simulink model "controller_simulation"  (R2017b)
settings: Solver=FixedStepAuto  StartTime=0.0  StopTime=10  FixedStep=0.01  RelTol=1e-3
values from neighbouring files (symbols this model uses):
  g = sym(zeros(length(d),1))    [kinematic_dynamic.m]    (also in simplifyG.m = g*49/5)
  m = [0 0 m1 0 0 0 0 m2]    [kinematic_dynamic.m]
libraries: simulink x6
settings Model: Creator=Ufuk  LastModifiedBy=Ufuk

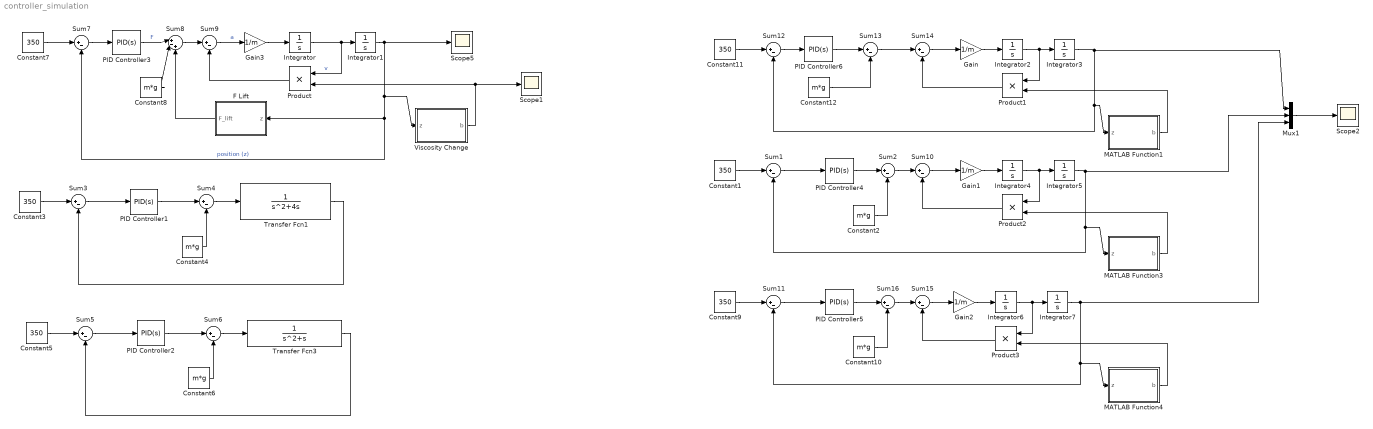
== system controller_simulation ==
  Constant{1,3,5,7,9,11} (6 alike) : Constant  Value=350
  Constant{2,4,6,8,10,12} (6 alike) : Constant  Value=m*g
  F Lift : MATLAB Function  TreatAsAtomicUnit=on
  Gain{,1..3} (4 alike) : Gain  Gain=1/m
  Integrator{,1..7} (8 alike) : Integrator
  MATLAB Function1 : MATLAB Function  TreatAsAtomicUnit=on
  MATLAB Function3 : MATLAB Function  TreatAsAtomicUnit=on
  MATLAB Function4 : MATLAB Function  TreatAsAtomicUnit=on
  Mux1 : Mux  Inputs=3
  PID Controller{1..3,6} (4 alike) : simulink/Continuous/PID Controller  Controller=PID  TimeDomain=Continuous-time  SampleTime=-1  IntegratorMethod=Forward Euler  FilterMethod=Forward Euler  Form=Parallel  UseFilter=on  ControllerParametersSource=internal  P=20  I=0  D=0  N=100  InitialConditionSource=internal  InitialConditionForIntegrator=0  InitialConditionForFilter=0  ExternalReset=none  LimitOutput=off  UpperSaturationLimit=inf  LowerSaturationLimit=-inf  LinearizeAsGain=on  AntiWindupMode=none  Kb=1  TrackingMode=off  Kt=1  PParamMin=[]  PParamMax=[]  IParamMin=[]  IParamMax=[]  DParamMin=[]  DParamMax=[]  NParamMin=[]  NParamMax=[]  KbParamMin=[]  KbParamMax=[]  KtParamMin=[]  KtParamMax=[]  POutMin=[]  POutMax=[]  IOutMin=[]  IOutMax=[]  DOutMin=[]  DOutMax=[]  NOutMin=[]  NOutMax=[]  KbOutMin=[]  KbOutMax=[]  KtOutMin=[]  KtOutMax=[]  IntegratorOutMin=[]  IntegratorOutMax=[]  FilterOutMin=[]  FilterOutMax=[]  SumOutMin=[]  SumOutMax=[]  SumI1OutMin=[]  SumI1OutMax=[]  SumI2OutMin=[]  SumI2OutMax=[]  SumI3OutMin=[]  SumI3OutMax=[]  SumDOutMin=[]  SumDOutMax=[]  SaturationOutMin=[]  SaturationOutMax=[]  IntegratorContinuousStateAttributes=''  IntegratorStateMustResolveToSignalObject=off  IntegratorRTWStateStorageClass=Auto  FilterContinuousStateAttributes=''  FilterStateMustResolveToSignalObject=off  FilterRTWStateStorageClass=Auto  DifferentiatorICPrevScaledInput=0  DifferentiatorOutMin=[]  DifferentiatorOutMax=[]  InitialConditionSetting=State (most efficient)  FilterDiffOutCoefMin=[]  FilterDiffOutCoefMax=[]  SumDenOutMin=[]  SumDenOutMax=[]  SumNumOutMin=[]  SumNumOutMax=[]  ReciprocalOutMin=[]  ReciprocalOutMax=[]  DivideOutMin=[]  DivideOutMax=[]  TunerSelectOption=Transfer Function Based (PID Tuner App)
  PID Controller4 : simulink/Continuous/PID Controller  Controller=PID  TimeDomain=Continuous-time  SampleTime=-1  IntegratorMethod=Forward Euler  FilterMethod=Forward Euler  Form=Parallel  UseFilter=on  ControllerParametersSource=internal  P=15  I=2  D=0  N=100  InitialConditionSource=internal  InitialConditionForIntegrator=0  InitialConditionForFilter=0  ExternalReset=none  LimitOutput=off  UpperSaturationLimit=inf  LowerSaturationLimit=-inf  LinearizeAsGain=on  AntiWindupMode=none  Kb=1  TrackingMode=off  Kt=1  PParamMin=[]  PParamMax=[]  IParamMin=[]  IParamMax=[]  DParamMin=[]  DParamMax=[]  NParamMin=[]  NParamMax=[]  KbParamMin=[]  KbParamMax=[]  KtParamMin=[]  KtParamMax=[]  POutMin=[]  POutMax=[]  IOutMin=[]  IOutMax=[]  DOutMin=[]  DOutMax=[]  NOutMin=[]  NOutMax=[]  KbOutMin=[]  KbOutMax=[]  KtOutMin=[]  KtOutMax=[]  IntegratorOutMin=[]  IntegratorOutMax=[]  FilterOutMin=[]  FilterOutMax=[]  SumOutMin=[]  SumOutMax=[]  SumI1OutMin=[]  SumI1OutMax=[]  SumI2OutMin=[]  SumI2OutMax=[]  SumI3OutMin=[]  SumI3OutMax=[]  SumDOutMin=[]  SumDOutMax=[]  SaturationOutMin=[]  SaturationOutMax=[]  IntegratorContinuousStateAttributes=''  IntegratorStateMustResolveToSignalObject=off  IntegratorRTWStateStorageClass=Auto  FilterContinuousStateAttributes=''  FilterStateMustResolveToSignalObject=off  FilterRTWStateStorageClass=Auto  DifferentiatorICPrevScaledInput=0  DifferentiatorOutMin=[]  DifferentiatorOutMax=[]  InitialConditionSetting=State (most efficient)  FilterDiffOutCoefMin=[]  FilterDiffOutCoefMax=[]  SumDenOutMin=[]  SumDenOutMax=[]  SumNumOutMin=[]  SumNumOutMax=[]  ReciprocalOutMin=[]  ReciprocalOutMax=[]  DivideOutMin=[]  DivideOutMax=[]  TunerSelectOption=Transfer Function Based (PID Tuner App)
  PID Controller5 : simulink/Continuous/PID Controller  Controller=PID  TimeDomain=Continuous-time  SampleTime=-1  IntegratorMethod=Forward Euler  FilterMethod=Forward Euler  Form=Parallel  UseFilter=on  ControllerParametersSource=internal  P=15  I=2  D=1  N=100  InitialConditionSource=internal  InitialConditionForIntegrator=0  InitialConditionForFilter=0  ExternalReset=none  LimitOutput=off  UpperSaturationLimit=inf  LowerSaturationLimit=-inf  LinearizeAsGain=on  AntiWindupMode=none  Kb=1  TrackingMode=off  Kt=1  PParamMin=[]  PParamMax=[]  IParamMin=[]  IParamMax=[]  DParamMin=[]  DParamMax=[]  NParamMin=[]  NParamMax=[]  KbParamMin=[]  KbParamMax=[]  KtParamMin=[]  KtParamMax=[]  POutMin=[]  POutMax=[]  IOutMin=[]  IOutMax=[]  DOutMin=[]  DOutMax=[]  NOutMin=[]  NOutMax=[]  KbOutMin=[]  KbOutMax=[]  KtOutMin=[]  KtOutMax=[]  IntegratorOutMin=[]  IntegratorOutMax=[]  FilterOutMin=[]  FilterOutMax=[]  SumOutMin=[]  SumOutMax=[]  SumI1OutMin=[]  SumI1OutMax=[]  SumI2OutMin=[]  SumI2OutMax=[]  SumI3OutMin=[]  SumI3OutMax=[]  SumDOutMin=[]  SumDOutMax=[]  SaturationOutMin=[]  SaturationOutMax=[]  IntegratorContinuousStateAttributes=''  IntegratorStateMustResolveToSignalObject=off  IntegratorRTWStateStorageClass=Auto  FilterContinuousStateAttributes=''  FilterStateMustResolveToSignalObject=off  FilterRTWStateStorageClass=Auto  DifferentiatorICPrevScaledInput=0  DifferentiatorOutMin=[]  DifferentiatorOutMax=[]  InitialConditionSetting=State (most efficient)  FilterDiffOutCoefMin=[]  FilterDiffOutCoefMax=[]  SumDenOutMin=[]  SumDenOutMax=[]  SumNumOutMin=[]  SumNumOutMax=[]  ReciprocalOutMin=[]  ReciprocalOutMax=[]  DivideOutMin=[]  DivideOutMax=[]  TunerSelectOption=Transfer Function Based (PID Tuner App)
  Product{,1..3} (4 alike) : Product
  Scope1 : Scope
  Scope2 : Scope
  Scope5 : Scope
  Sum{1..7,9..16} (15 alike) : Sum  Inputs=|+-
  Sum8 : Sum  Inputs=|+-+
  Transfer Fcn1 : TransferFcn  Denominator=[1 4 0]
  Transfer Fcn3 : TransferFcn  Denominator=[1 1 0]
  Viscosity Change : MATLAB Function  TreatAsAtomicUnit=on
  wires:
  Transfer Fcn1/1 -> Sum3/2
  Product/1 -> Sum9/2
  Sum6/1 -> Transfer Fcn3/1
  PID Controller2/1 -> Sum6/1
  Sum5/1 -> PID Controller2/1
  Viscosity Change/1(b) -> Product/2, Scope1/1
  Sum8/1 -> Sum9/1
  Integrator/1 -> Product/1, Integrator1/1  "v"
  Sum9/1 -> Gain3/1  "a"
  Integrator1/1 -> Scope5/1, F Lift/1(z), Sum7/2, Viscosity Change/1(z)  "position (z)"
  Sum3/1 -> PID Controller1/1
  Sum7/1 -> PID Controller3/1
  Constant6/1 -> Sum6/2
  Constant8/1 -> Sum8/2
  Constant3/1 -> Sum3/1
  PID Controller1/1 -> Sum4/1
  Constant4/1 -> Sum4/2
  Constant7/1 -> Sum7/1
  Sum4/1 -> Transfer Fcn1/1
  Transfer Fcn3/1 -> Sum5/2
  PID Controller3/1 -> Sum8/1  "F"
  Constant5/1 -> Sum5/1
  MATLAB Function1/1(b) -> Product1/2
  Constant12/1 -> Sum13/2
  Sum13/1 -> Sum14/1
  Product1/1 -> Sum14/2
  Integrator2/1 -> Product1/1, Integrator3/1
  Integrator3/1 -> Mux1/1, MATLAB Function1/1(z), Sum12/2
  Mux1/1 -> Scope2/1
  Sum12/1 -> PID Controller6/1
  Constant11/1 -> Sum12/1
  PID Controller6/1 -> Sum13/1
  Sum14/1 -> Gain/1
  PID Controller4/1 -> Sum2/1
  Constant1/1 -> Sum1/1
  Sum1/1 -> PID Controller4/1
  Integrator5/1 -> Mux1/2, MATLAB Function3/1(z), Sum1/2
  Integrator4/1 -> Product2/1, Integrator5/1
  Product2/1 -> Sum10/2
  MATLAB Function3/1(b) -> Product2/2
  Sum2/1 -> Sum10/1
  Sum10/1 -> Gain1/1
  Constant2/1 -> Sum2/2
  Sum15/1 -> Gain2/1
  Sum16/1 -> Sum15/1
  MATLAB Function4/1(b) -> Product3/2
  Product3/1 -> Sum15/2
  Integrator6/1 -> Product3/1, Integrator7/1
  Integrator7/1 -> Mux1/3, MATLAB Function4/1(z), Sum11/2
  Constant10/1 -> Sum16/2
  Sum11/1 -> PID Controller5/1
  PID Controller5/1 -> Sum16/1
  Constant9/1 -> Sum11/1
  Gain/1 -> Integrator2/1
  Gain1/1 -> Integrator4/1
  Gain2/1 -> Integrator6/1
  Gain3/1 -> Integrator/1
  F Lift/1(F_lift) -> Sum8/3

== matlab function controller_simulation/MATLAB Function1 ==
  data: z input; b output
function b = fcn(z)
b_water=4,;
b_air=1;
b_mixed=b_water*(100-(z-300))/100+b_air*(z-300)/100

if z<=300
b = b_water;
elseif (z<=400) && (300<=z)
b = b_mixed;
else
b = b_air;
end

== matlab function controller_simulation/Viscosity Change ==
  data: z input; b output
function b = fcn(z)
b_water=4,;
b_air=1;
b_mixed=b_water*(100-(z-300))/100+b_air*(z-300)/100

if z<=300
b = b_water;
elseif (z<=400) && (300<=z)
b = b_mixed;
else
b = b_air;
end

== matlab function controller_simulation/MATLAB Function3 ==
  data: z input; b output
function b = fcn(z)
b_water=4,;
b_air=1;
b_mixed=b_water*(100-(z-300))/100+b_air*(z-300)/100

if z<=300
b = b_water;
elseif (z<=400) && (300<=z)
b = b_mixed;
else
b = b_air;
end

== matlab function controller_simulation/MATLAB Function4 ==
  data: z input; b output
function b = fcn(z)
b_water=4,;
b_air=1;
b_mixed=b_water*(100-(z-300))/100+b_air*(z-300)/100

if z<=300
b = b_water;
elseif (z<=400) && (300<=z)
b = b_mixed;
else
b = b_air;
end

== matlab function controller_simulation/F Lift ==
  data: z input; F_lift output
function F_lift = fcn(z)
k=1;
F_lift=k*(100-(z-300))/100;
